simulink model "P2_d"  (R2024a)
settings: Solver=VariableStepAuto  StartTime=0.0  StopTime=10.0  RelTol=1e-3
libraries: simulink x1
settings Model: Creator=Rajatsurya  LastModifiedBy=Rajatsurya

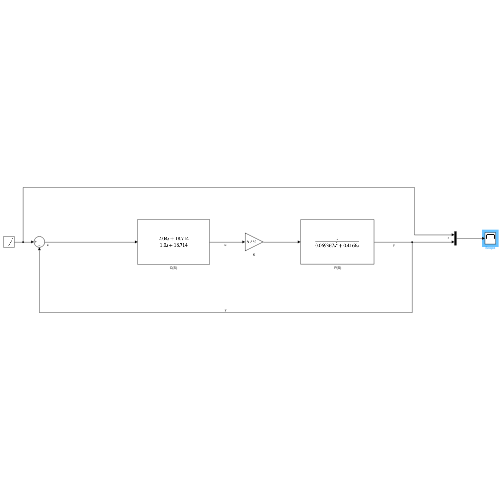
[thumbnail: Simulink's stored preview of the top-level diagram]
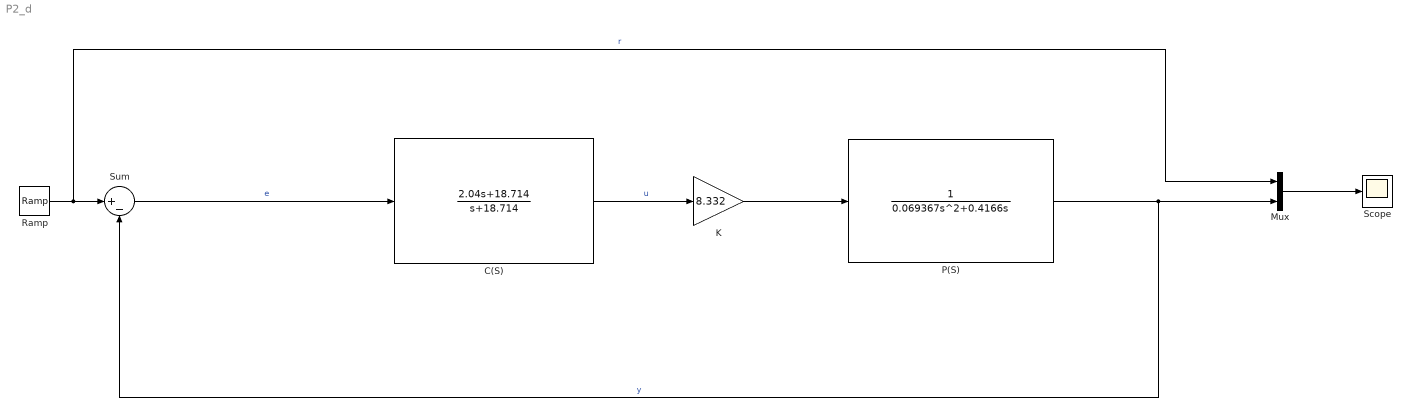
== system P2_d ==
  " P(S)" : TransferFcn  Denominator=[0.069367 0.4166 0]
  C(S) : TransferFcn  Numerator=[2.04 18.714]  Denominator=[1.0 18.714 ]
  K : Gain  Gain=8.332
  Mux : Mux  Inputs=2
  Ramp : simulink/Sources/Ramp  slope=1  start=0  InitialOutput=0
  Scope : Scope
  Sum : Sum  Inputs=|+-
  wires:
  " P(S)"/1 -> Mux/2, Sum/2  "y"
  C(S)/1 -> K/1  "u"
  Ramp/1 -> Mux/1, Sum/1  "r"
  Mux/1 -> Scope/1
  Sum/1 -> C(S)/1  "e"
  K/1 -> " P(S)"/1
